simulink subsystem "Torque_Vectoring_2WD_NO_FILTER_NO_REGEN"  (R2023b)
settings: Solver=VariableStepAuto  StartTime=0.0  StopTime=10.0  RelTol=1e-3
undefined symbols (not defined in the file): bI_bias, bI_gain, bT_bias, bT_gain, half_track, mcT_bias, mcT_gain, mT_bias, mT_gain, r_power_sat, rb, s, v, yaw_table
libraries: simulink x2
settings Model: Creator=Inver  LastModifiedBy=Inver
settings SFSimCC: SimCustomHeaderCode="#include \"simplex.h\""  SimUserSources=Code_Generation_Project/simplex.c

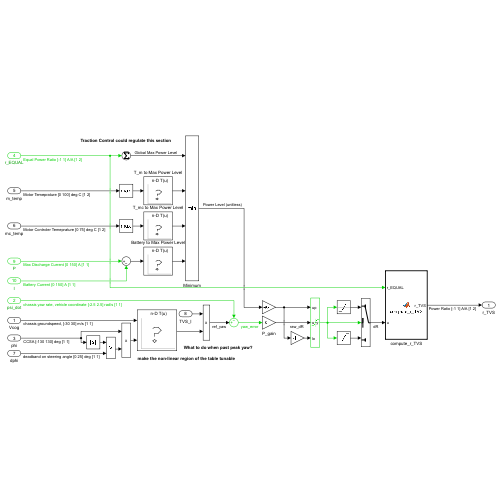
[thumbnail: Simulink's stored preview of the top-level diagram]
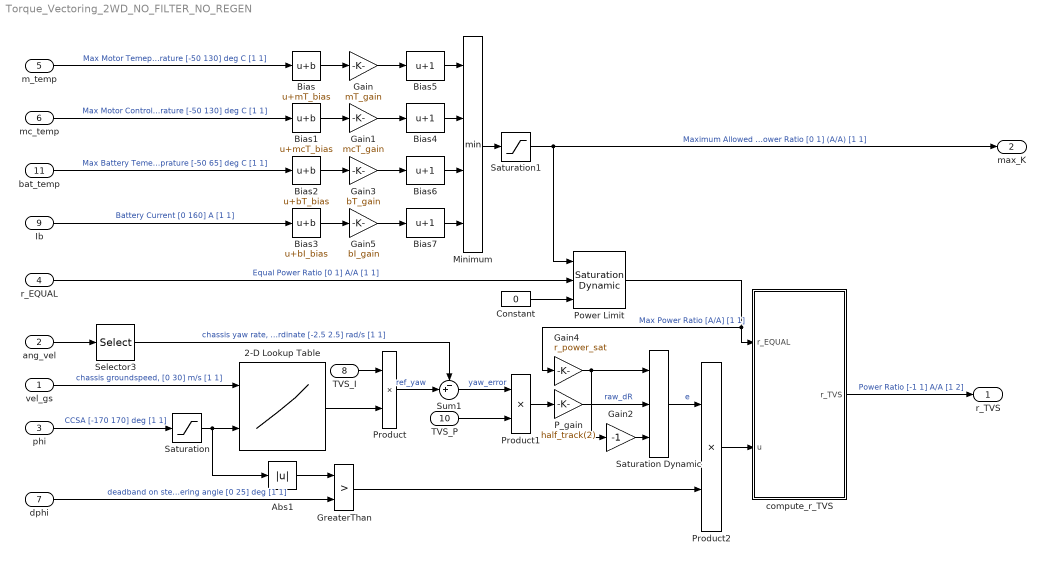
== system Torque_Vectoring_2WD_NO_FILTER_NO_REGEN ==
  vel_gs : Inport
  ang_vel : Inport  Port=2  OutDataTypeStr=double  LockScale=on
  phi : Inport  Port=3
  r_EQUAL : Inport  Port=4  OutDataTypeStr=double  LockScale=on
  m_temp : Inport  Port=5
  mc_temp : Inport  Port=6
  dphi : Inport  Port=7
  TVS_I : Inport  Port=8
  Ib : Inport  Port=9  OutDataTypeStr=double  LockScale=on
  TVS_P : Inport  Port=10
  bat_temp : Inport  Port=11
  2-D Lookup Table : Lookup_n-D  BreakpointsForDimension1=v  BreakpointsForDimension2=s  IndexSearchMethod=Evenly spaced points  Table=yaw_table  ExtrapMethod=Clip  UseLastTableValue=on  InternalRulePriority=Speed  RndMeth=Simplest
      settings: InputPortMap=u0,u1
  Abs1 : Abs  SaturateOnIntegerOverflow=off
  Bias : Bias  Bias=mT_bias  SaturateOnIntegerOverflow=off
  Bias1 : Bias  Bias=mcT_bias  SaturateOnIntegerOverflow=off
  Bias2 : Bias  Bias=bT_bias  SaturateOnIntegerOverflow=off
  Bias3 : Bias  Bias=bI_bias  SaturateOnIntegerOverflow=off
  Bias{4..7} (4 alike) : Bias  Bias=1  SaturateOnIntegerOverflow=off
  Constant : Constant  Value=0
  Gain : Gain  Gain=mT_gain
  Gain1 : Gain  Gain=mcT_gain
  Gain2 : Gain  Gain=-1
  Gain3 : Gain  Gain=bT_gain
  Gain4 : Gain  Gain=r_power_sat
  Gain5 : Gain  Gain=bI_gain
  GreaterThan : RelationalOperator  Operator=>  OutDataTypeStr=boolean  RndMeth=Simplest  InputSameDT=off
  Minimum : MinMax  Inputs=4
  P_gain : Gain  Gain=half_track(2)  ParamDataTypeStr=double  OutDataTypeStr=double
  Power Limit : simulink/Discontinuities/Saturation Dynamic  OutMin=[]  OutMax=[]  OutDataTypeStr=Inherit: Same as second input  OutDataType=fixdt(1, 16)  OutScaling=2^-10  DoSatur=off
  Product : Product  OutDataTypeStr=Inherit: Inherit via back propagation
  Product1 : Product
  Product2 : Product
  Saturation : Saturate  UpperLimit=130  LowerLimit=-130
  Saturation Dynamic : simulink/Discontinuities/Saturation Dynamic  OutMin=[]  OutMax=[]  OutDataTypeStr=Inherit: Same as second input  OutDataType=fixdt(1, 16)  OutScaling=2^-10  DoSatur=off
  Saturation1 : Saturate  UpperLimit=rb(2)  LowerLimit=rb(1)
  Selector3 : Selector  IndexMode=Zero-based  InputPortWidth=3  IndexOptions=Index vector (dialog)  Indices=2  OutputSizes=1
  Sum1 : Sum  Inputs=-+|  OutDataTypeStr=Inherit: Inherit via back propagation
  compute_r_TVS : MATLAB Function  TreatAsAtomicUnit=on
  r_TVS : Outport
  max_K : Outport  Port=2
  wires:
  Ib/1 -> Bias3/1  "Battery Current [0 160] A [1 1]"
  Saturation/1 -> Abs1/1, 2-D Lookup Table/2
  phi/1 -> Saturation/1  "CCSA [-170 170] deg [1 1]"
  Saturation Dynamic/1 -> Product2/1  "e"
  m_temp/1 -> Bias/1  "Max Motor Temeprature [-50 130] deg C [1 1]"
  r_EQUAL/1 -> Power Limit/2  "Equal Power Ratio [0 1] A/A [1 1]"
  Power Limit/1 -> Gain4/1, compute_r_TVS/1(r_EQUAL)  "Max Power Ratio [A/A] [1 1]"
  vel_gs/1 -> 2-D Lookup Table/1  "chassis groundspeed, [0 30] m/s [1 1]"
  mc_temp/1 -> Bias1/1  "Max Motor Controler Temeprature [-50 130] deg C [1 1]"
  Bias1/1 -> Gain1/1
  Bias/1 -> Gain/1
  TVS_I/1 -> Product/1
  Product/1 -> Sum1/2  "ref_yaw"
  ang_vel/1 -> Selector3/1
  2-D Lookup Table/1 -> Product/2
  GreaterThan/1 -> Product2/2
  Abs1/1 -> GreaterThan/1
  Sum1/1 -> Product1/1  "yaw_error"
  Gain2/1 -> Saturation Dynamic/3
  Gain4/1 -> Saturation Dynamic/1, Gain2/1
  dphi/1 -> GreaterThan/2  "deadband on steering angle [0 25] deg [1 1]"
  P_gain/1 -> Saturation Dynamic/2  "raw_dR"
  compute_r_TVS/1(r_TVS) -> r_TVS/1  "Power Ratio [-1 1] A/A [1 2]"
  Selector3/1 -> Sum1/1  "chassis yaw rate, vehicle coordinate [-2.5 2.5] rad/s [1 1]"
  TVS_P/1 -> Product1/2
  Product1/1 -> P_gain/1
  Saturation1/1 -> max_K/1, Power Limit/1  "Maximum Allowed Power Ratio [0 1] (A/A) [1 1]"
  bat_temp/1 -> Bias2/1  "Max Battery Temeprature [-50 65] deg C [1 1]"
  Bias2/1 -> Gain3/1
  Bias3/1 -> Gain5/1
  Gain/1 -> Bias5/1
  Gain1/1 -> Bias4/1
  Gain3/1 -> Bias6/1
  Gain5/1 -> Bias7/1
  Bias5/1 -> Minimum/1
  Bias4/1 -> Minimum/2
  Bias6/1 -> Minimum/3
  Bias7/1 -> Minimum/4
  Minimum/1 -> Saturation1/1
  Constant/1 -> Power Limit/3
  Product2/1 -> compute_r_TVS/2(u)

== matlab function Torque_Vectoring_2WD_NO_FILTER_NO_REGEN/compute_r_TVS ==
  data: r_EQUAL input; u input; r_TVS output
function r_TVS = compute_r_TVS(r_EQUAL,u)
    if u > 0
        r_TVS = [r_EQUAL(1) r_EQUAL(1)-abs(u)];
    else
        r_TVS = [r_EQUAL(1)-abs(u) r_EQUAL(1)];
    end
end
